simulink model "openloop501"  (R2022a)
settings: Solver=VariableStepAuto  StartTime=0.0  StopTime=50000  RelTol=1e-3
settings Model: Creator=danie  LastModifiedBy=danie

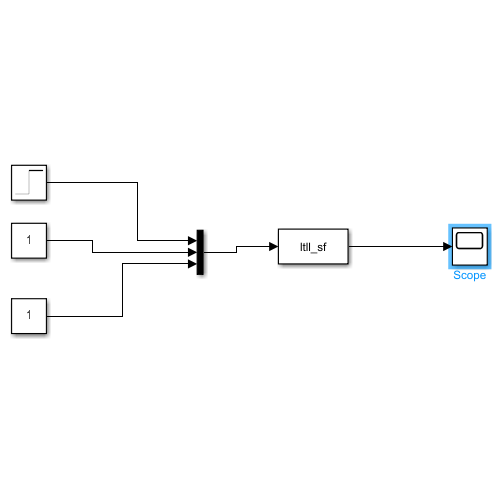
[thumbnail: Simulink's stored preview of the top-level diagram]
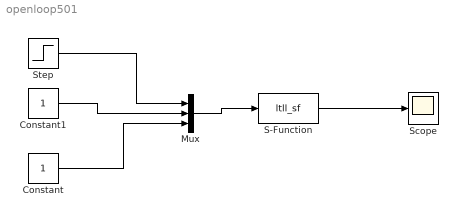
== system openloop501 ==
  Constant : Constant
  Constant1 : Constant
  Mux : Mux  Inputs=3
  S-Function : S-Function  FunctionName=ltll_sf  SFunctionDeploymentMode=off  EnableBusSupport=off
  Scope : Scope
  Step : Step  Time=0  Before=2.5  After=2.5  SampleTime=0
  wires:
  S-Function/1 -> Scope/1
  Step/1 -> Mux/1
  Constant1/1 -> Mux/2
  Constant/1 -> Mux/3
  Mux/1 -> S-Function/1
